simulink model "PEN1"  (R2018b)
settings: Solver=VariableStepAuto  StartTime=0.0  StopTime=10  RelTol=1e-3
settings Model: Creator=ohara  LastModifiedBy=ohara

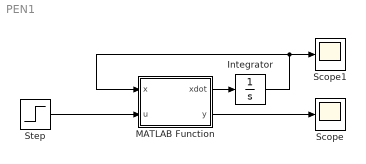
== system PEN1 ==
  Integrator : Integrator  InitialCondition=[3,0]
  MATLAB Function : MATLAB Function  TreatAsAtomicUnit=on
  Scope : Scope
  Scope1 : Scope
  Step : Step  SampleTime=0
  wires:
  Integrator/1 -> Scope1/1, MATLAB Function/1(x)
  MATLAB Function/1(xdot) -> Integrator/1
  MATLAB Function/2(y) -> Scope/1
  Step/1 -> MATLAB Function/2(u)

== matlab function PEN1/MATLAB Function ==
  data: x input; xdot output; u input; y output
function [xdot, y] = PEN(x, u)
a = 4;
b = 1;
gol = 12;
xdot1 = x(2);
xdot2 = gol*sin(x(1))-a*x(2)+b*u;
xdot  = [xdot1; xdot2];
y = x(1);
